simulink model "IID_nms_2Dmodel_inv"  (R2016b)
settings: Solver=ode3  StartTime=0.0  StopTime=tend  FixedStep=ts  RelTol=1e-3  EnableMultiTasking=on
InitFcn:
  | IID_runScripts_inv;
values from neighbouring files (symbols this model uses):
  DeltaThRef = 5e-3    (= 0.005)    [IID_nms_MechInit.m]    (also in nms_MechInit.m)
  MidDelay = 0.010    (= 0.01)    [IID_setCtrlPar.m]    (also in nms_MechInit.m = 0.005)
  ShortDelay = 0.005    [IID_setCtrlPar.m]    (also in nms_MechInit.m = 0.0025)
libraries: cpg_lib x18, simulink x11, simulink_extras x2
settings Model: SimulationMode=accelerator  Creator=Tycho  LastModifiedBy=brugtjh
settings DataIOCC: SignalLogging=off  SignalLoggingName=logout
settings OptimizationCC: LifeSpan=inf
settings DebuggingCC: AllowSymbolicDim=off  SFUnexpectedBacktrackingDiag=warning  SFNoUnconditionalDefaultTransitionDiag=warning  SFExecutionAtInitializationDiag=none
settings ModelReferenceCC: PropagateSignalLabelsOutOfModel=off
settings GRTTargetCC: TargetLangStandard=C89/C90 (ANSI)
settings ConfigComp: CovMetricSettings=dw  CovHtmlReporting=on  CovSaveCumulativeToWorkspaceVar=on  CovSaveSingleToWorkspaceVar=on  CovExternalEMLEnable=off

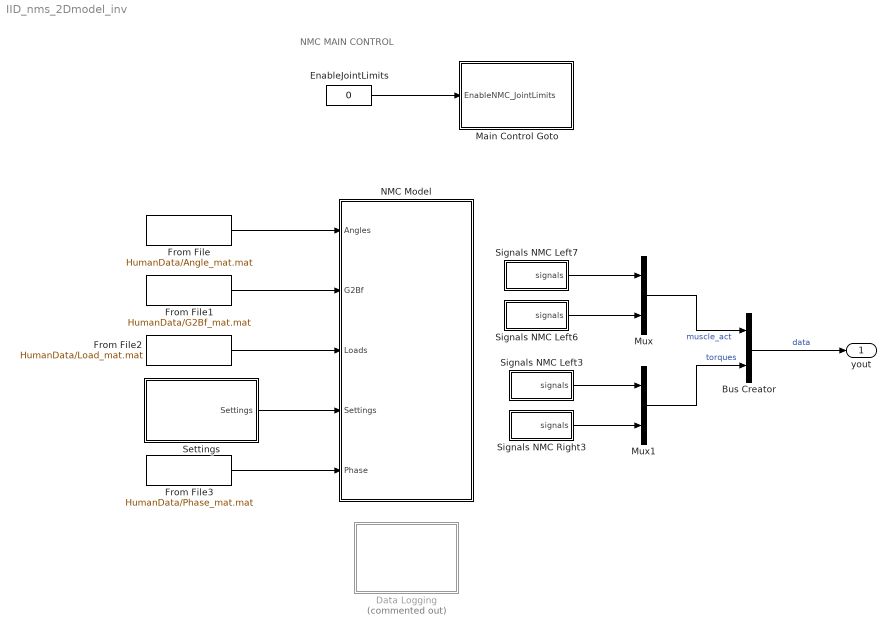
== system IID_nms_2Dmodel_inv ==
  note: NMC MAIN CONTROL
  Bus Creator : BusCreator  Inputs=2
  Data Logging : Subsystem  Commented=on
  EnableJointLimits : Constant  Value=0  OutDataTypeStr=double
      settings: OpenFcn=|
      | b = get_param(gcb,'value');
      | if (strcmp(b,'1')),
      |   set_param (gcb,'value','0');
      | else
      |   set_param(gcb,'value','1');
      | end;
  From File : FromFile  FileName=HumanData/Angle_mat.mat  SampleTime=0
  From File1 : FromFile  FileName=HumanData/G2Bf_mat.mat  SampleTime=0
  From File2 : FromFile  FileName=HumanData/Load_mat.mat  SampleTime=0
  From File3 : FromFile  FileName=HumanData/Phase_mat.mat  SampleTime=0
  Main Control Goto : Subsystem
  Mux : Mux  Inputs=2
  Mux1 : Mux  Inputs=2
  NMC Model : Subsystem
  Settings : Subsystem
  Signals NMC Left3 : Subsystem
  Signals NMC Left6 : Subsystem
  Signals NMC Left7 : Subsystem
  Signals NMC Right3 : Subsystem
  yout : Outport
  wires:
  Settings/1(Settings) -> NMC Model/4(Settings)
  EnableJointLimits/1 -> Main Control Goto/1(EnableNMC_JointLimits)
  From File/1 -> NMC Model/1(Angles)
  From File1/1 -> NMC Model/2(G2Bf)
  From File2/1 -> NMC Model/3(Loads)
  From File3/1 -> NMC Model/5(Phase)
  Signals NMC Left6/1(signals) -> Mux/2
  Signals NMC Left7/1(signals) -> Mux/1
  Signals NMC Left3/1(signals) -> Mux1/1
  Signals NMC Right3/1(signals) -> Mux1/2
  Mux/1 -> Bus Creator/1  "muscle_act"
  Mux1/1 -> Bus Creator/2  "torques"
  Bus Creator/1 -> yout/1  "data"

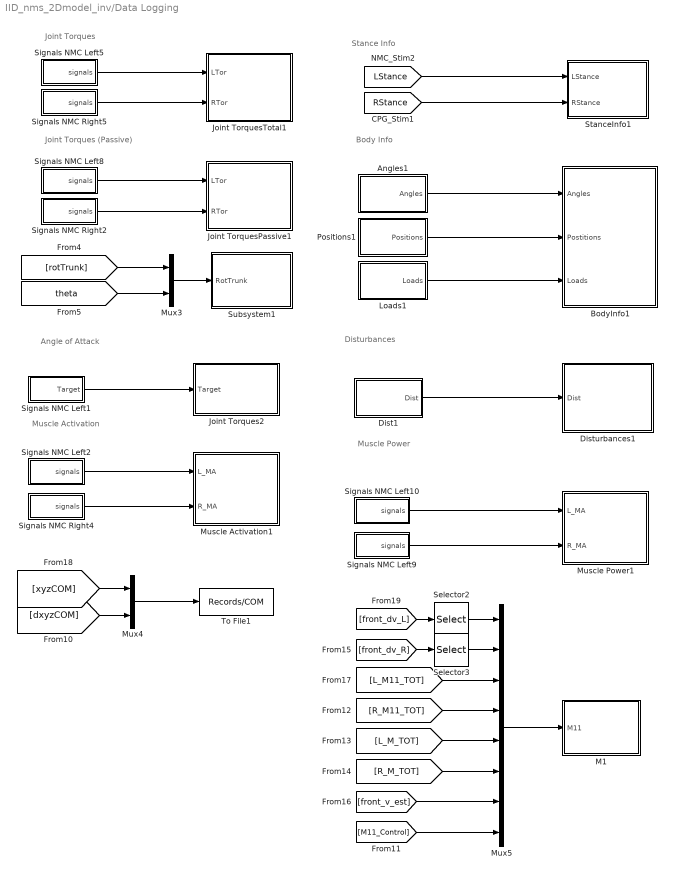
== system IID_nms_2Dmodel_inv/Data Logging ==
  note: Disturbances
  note: Stance Info
  note: Muscle Activation
  note: Joint Torques
  note: Angle of Attack
  note: Body Info
  note: Joint Torques (Passive)
  note: Muscle Power
  Angles1 : Subsystem
  BodyInfo1 : Subsystem
  Dist1 : Subsystem
  Disturbances1 : Subsystem
  Joint Torques2 : Subsystem
  Joint TorquesPassive1 : Subsystem
  Joint TorquesTotal1 : Subsystem
  Loads1 : Subsystem
  M1 : Subsystem
  Muscle Activation1 : Subsystem
  Muscle Power1 : Subsystem
  Mux3 : Mux  Inputs=2
  Mux4 : Mux  Inputs=2
  Mux5 : Mux  Inputs=8
  Positions1 : Subsystem
  Selector2 : Selector  InputPortWidth=2  IndexOptions=Index vector (dialog)  Indices=[2]  OutputSizes=1
  Selector3 : Selector  InputPortWidth=2  IndexOptions=Index vector (dialog)  Indices=[2]  OutputSizes=1
  Signals NMC Left1 : Subsystem
  Signals NMC Left10 : Subsystem
  Signals NMC Left2 : Subsystem
  Signals NMC Left5 : Subsystem
  Signals NMC Left8 : Subsystem
  Signals NMC Left9 : Subsystem
  Signals NMC Right2 : Subsystem
  Signals NMC Right4 : Subsystem
  Signals NMC Right5 : Subsystem
  StanceInfo1 : Subsystem
  Subsystem1 : Subsystem
  To File1 : ToFile  Filename=Records/COM
  wires:
  Dist1/1(Dist) -> Disturbances1/1(Dist)
  Signals NMC Right4/1(signals) -> Muscle Activation1/2(R_MA)
  Signals NMC Left2/1(signals) -> Muscle Activation1/1(L_MA)
  Signals NMC Left5/1(signals) -> Joint TorquesTotal1/1(LTor)
  Signals NMC Right5/1(signals) -> Joint TorquesTotal1/2(RTor)
  Angles1/1(Angles) -> BodyInfo1/1(Angles)
  Positions1/1(Positions) -> BodyInfo1/2(Postitions)
  [LStance] -> StanceInfo1/1(LStance)
  [RStance] -> StanceInfo1/2(RStance)
  Loads1/1(Loads) -> BodyInfo1/3(Loads)
  Signals NMC Left1/1(Target) -> Joint Torques2/1(Target)
  [rotTrunk] -> Mux3/1
  [theta] -> Mux3/2
  Signals NMC Left8/1(signals) -> Joint TorquesPassive1/1(LTor)
  Signals NMC Right2/1(signals) -> Joint TorquesPassive1/2(RTor)
  Signals NMC Left9/1(signals) -> Muscle Power1/2(R_MA)
  Signals NMC Left10/1(signals) -> Muscle Power1/1(L_MA)
  Mux3/1 -> Subsystem1/1(RotTrunk)
  [dxyzCOM] -> Mux4/2
  [xyzCOM] -> Mux4/1
  Mux4/1 -> To File1/1
  Selector2/1 -> Mux5/1
  [front_dv_L] -> Selector2/1
  [L_M_TOT] -> Mux5/5
  [R_M_TOT] -> Mux5/6
  [L_M11_TOT] -> Mux5/3
  [R_M11_TOT] -> Mux5/4
  [front_dv_R] -> Selector3/1
  Selector3/1 -> Mux5/2
  Mux5/1 -> M1/1(M11)
  [M11_Control] -> Mux5/8
  [front_v_est] -> Mux5/7

== system IID_nms_2Dmodel_inv/Main Control Goto ==
  EnableNMC_JointLimits : Inport
  tag scope: DisableNMC_JointLimitsIn=global
  wires:
  EnableNMC_JointLimits/1 -> [DisableNMC_JointLimitsIn]

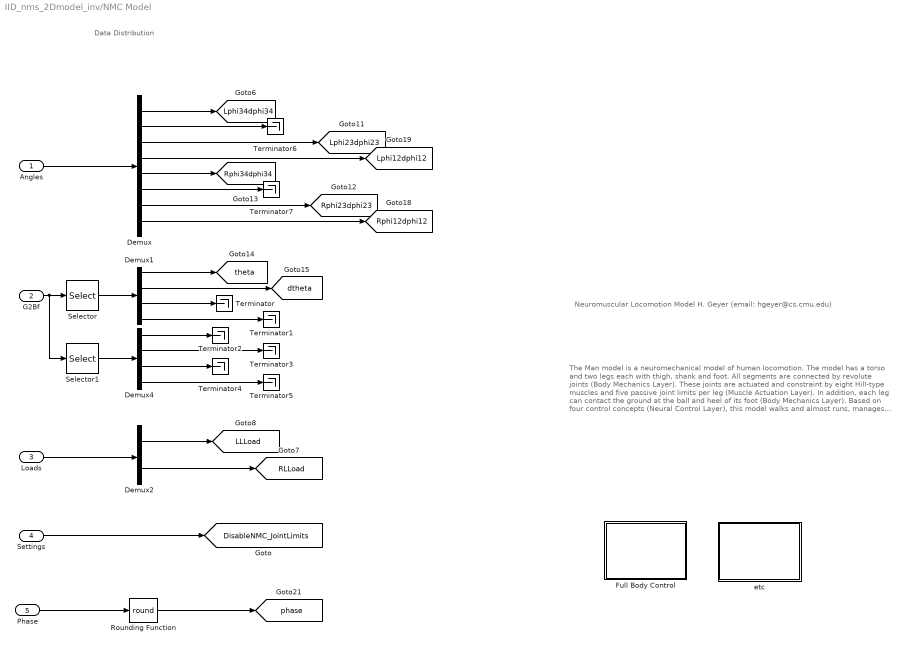
== system IID_nms_2Dmodel_inv/NMC Model ==
  note: Data Distribution
  note: The Man model is a neuromechanical model of human locomotion.
      | The model has a torso and two legs each with thigh, shank and
      | foot. All segments are connected by revolute joints (Body Mechanics
      | Layer). These joints are actuated and constraint by eight Hill-type
      | muscles and five passive joint limits per leg (Muscle Actuation Layer).
      | In addition, each leg can contact the ground at the ball and heel of
      | its foot (Body Mechanics Layer).
      |
      | Based on four control concepts (Neural Control Layer), this
      | model walks and almost runs, manages slopes and random ground
      | levels, and adapts to different surfaces.
  note: Neuromuscular Locomotion Model
      | H. Geyer
      | (email: hgeyer@cs.cmu.edu)
  Angles : Inport
  G2Bf : Inport  Port=2
  Loads : Inport  Port=3
  Settings : Inport  Port=4
  Phase : Inport  Port=5
  Demux : Demux  Outputs=8
  Demux1 : Demux
  Demux2 : Demux  Outputs=2
  Demux4 : Demux
  Full Body Control : Subsystem
  Rounding Function : Rounding  Operator=round
  Selector : Selector  InputPortWidth=12  IndexOptions=Index vector (dialog)  Indices=[1:4]  OutputSizes=1
  Selector1 : Selector  InputPortWidth=12  IndexOptions=Index vector (dialog)  Indices=[5:12]  OutputSizes=1
  Terminator{,1..7} (8 alike) : Terminator
  etc : Subsystem
  tag scope: DisableNMC_JointLimits=global, LLLoad=global, Lphi12dphi12=global, Lphi23dphi23=global, Lphi34dphi34=global, RLLoad=global, Rphi12dphi12=global, Rphi23dphi23=global, Rphi34dphi34=global, dtheta=global, phase=global, theta=global
  wires:
  Settings/1 -> [DisableNMC_JointLimits]
  Phase/1 -> Rounding Function/1
  Loads/1 -> Demux2/1
  G2Bf/1 -> Selector1/1, Selector/1
  Demux/4 -> [Lphi12dphi12]
  Demux/3 -> [Lphi23dphi23]
  Demux/2 -> Terminator6/1
  Demux/8 -> [Rphi12dphi12]
  Demux/7 -> [Rphi23dphi23]
  Demux/6 -> Terminator7/1
  Demux/5 -> [Rphi34dphi34]
  Demux/1 -> [Lphi34dphi34]
  Angles/1 -> Demux/1
  Demux1/4 -> Terminator1/1
  Demux1/3 -> Terminator/1
  Demux1/2 -> [dtheta]
  Demux1/1 -> [theta]
  Selector/1 -> Demux1/1
  Selector1/1 -> Demux4/1
  Rounding Function/1 -> [phase]
  Demux4/1 -> Terminator2/1
  Demux4/3 -> Terminator4/1
  Demux4/2 -> Terminator3/1
  Demux4/4 -> Terminator5/1
  Demux2/1 -> [LLLoad]
  Demux2/2 -> [RLLoad]

== system IID_nms_2Dmodel_inv/Settings ==
  Settings : Outport
  wires:
  [DisableNMC_JointLimitsIn] -> Settings/1

== system IID_nms_2Dmodel_inv/Signals NMC Left3 ==
  Mux : Mux
  signals : Outport
  wires:
  Mux/1 -> signals/1
  [LM34] -> Mux/1
  [LM23] -> Mux/3
  [LM12] -> Mux/4
  [LM34R] -> Mux/2

== system IID_nms_2Dmodel_inv/Signals NMC Left6 ==
  Mux : Mux  Inputs=7
  signals : Outport
  wires:
  Mux/1 -> signals/1
  [REnergyVAS] -> Mux/2
  [REnergyHFL] -> Mux/1
  [REnergyTA] -> Mux/3
  [REnergySOL] -> Mux/4
  [REnergyHAM] -> Mux/6
  [REnergyGAS] -> Mux/5
  [REnergyGLU] -> Mux/7

== system IID_nms_2Dmodel_inv/Signals NMC Left7 ==
  Mux : Mux  Inputs=7
  signals : Outport
  wires:
  Mux/1 -> signals/1
  [LEnergyVAS] -> Mux/2
  [LEnergyHFL] -> Mux/1
  [LEnergyTA] -> Mux/3
  [LEnergySOL] -> Mux/4
  [LEnergyHAM] -> Mux/6
  [LEnergyGAS] -> Mux/5
  [LEnergyGLU] -> Mux/7

== system IID_nms_2Dmodel_inv/Signals NMC Right3 ==
  Mux : Mux
  signals : Outport
  wires:
  Mux/1 -> signals/1
  [RM34] -> Mux/1
  [RM23] -> Mux/3
  [RM12] -> Mux/4
  [RM34R] -> Mux/2

== system IID_nms_2Dmodel_inv/Data Logging/Angles1 ==
  Constant : Constant  Value=zeros(2,1)
  Constant1 : Constant  Value=zeros(2,1)
  Mux : Mux  Inputs=8
  Angles : Outport
  wires:
  [Rphi12dphi12] -> Mux/8
  [Lphi34dphi34] -> Mux/1
  [Rphi23dphi23] -> Mux/7
  [Lphi23dphi23] -> Mux/3
  Constant1/1 -> Mux/6
  Constant/1 -> Mux/2
  [Lphi12dphi12] -> Mux/4
  [Rphi34dphi34] -> Mux/5
  Mux/1 -> Angles/1

== system IID_nms_2Dmodel_inv/Data Logging/BodyInfo1 ==
  Angles : Inport
  Postitions : Inport  Port=2
  Loads : Inport  Port=3
  Mux1 : Mux  Inputs=3
  To File8 : ToFile  Filename=Records/BodyInfo
  wires:
  Loads/1 -> Mux1/3
  Postitions/1 -> Mux1/2
  Mux1/1 -> To File8/1
  Angles/1 -> Mux1/1

== system IID_nms_2Dmodel_inv/Data Logging/Dist1 ==
  Dist : Outport
  wires:
  [xyzHAT_D_sag] -> Dist/1

== system IID_nms_2Dmodel_inv/Data Logging/Disturbances1 ==
  Dist : Inport
  To File21 : ToFile  Filename=Records/Disturbance
  wires:
  Dist/1 -> To File21/1

== system IID_nms_2Dmodel_inv/Data Logging/Joint Torques2 ==
  Target : Inport
  To File12 : ToFile  Filename=Records/TargetAngle
  wires:
  Target/1 -> To File12/1

== system IID_nms_2Dmodel_inv/Data Logging/Joint TorquesPassive1 ==
  LTor : Inport
  RTor : Inport  Port=2
  To File12 : ToFile  Filename=Records/L_Tor_Passive
  To File9 : ToFile  Filename=Records/R_Tor_Passvie
  wires:
  RTor/1 -> To File9/1
  LTor/1 -> To File12/1

== system IID_nms_2Dmodel_inv/Data Logging/Joint TorquesTotal1 ==
  LTor : Inport
  RTor : Inport  Port=2
  To File12 : ToFile  Filename=Records/L_Tor
  To File9 : ToFile  Filename=Records/R_Tor
  wires:
  LTor/1 -> To File12/1
  RTor/1 -> To File9/1

== system IID_nms_2Dmodel_inv/Data Logging/Loads1 ==
  Mux : Mux  Inputs=2
  Loads : Outport
  wires:
  [LLLoad] -> Mux/2
  [RLLoad] -> Mux/1
  Mux/1 -> Loads/1

== system IID_nms_2Dmodel_inv/Data Logging/M1 ==
  M11 : Inport
  To File2 : ToFile  Filename=Records/M11
  wires:
  M11/1 -> To File2/1

== system IID_nms_2Dmodel_inv/Data Logging/Muscle Activation1 ==
  L_MA : Inport
  R_MA : Inport  Port=2
  To File1 : ToFile  Filename=Records/R_MA
  To File5 : ToFile  Filename=Records/L_MA
  wires:
  L_MA/1 -> To File5/1
  R_MA/1 -> To File1/1

== system IID_nms_2Dmodel_inv/Data Logging/Muscle Power1 ==
  L_MA : Inport
  R_MA : Inport  Port=2
  To File1 : ToFile  Filename=Records/R_Power
  To File5 : ToFile  Filename=Records/L_Power
  wires:
  L_MA/1 -> To File5/1
  R_MA/1 -> To File1/1

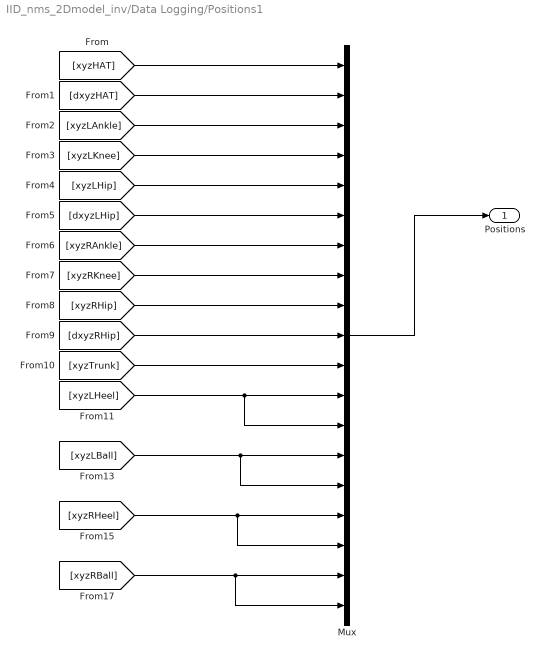
== system IID_nms_2Dmodel_inv/Data Logging/Positions1 ==
  Mux : Mux  Inputs=19
  Positions : Outport
  wires:
  [xyzRBall] -> Mux/19, Mux/18
  [xyzRHeel] -> Mux/17, Mux/16
  [xyzLBall] -> Mux/15, Mux/14
  [xyzLHeel] -> Mux/13, Mux/12
  [xyzTrunk] -> Mux/11
  [dxyzHAT] -> Mux/2
  [xyzHAT] -> Mux/1
  [dxyzRHip] -> Mux/10
  [xyzRHip] -> Mux/9
  [xyzLAnkle] -> Mux/3
  [xyzRKnee] -> Mux/8
  [dxyzLHip] -> Mux/6
  [xyzLHip] -> Mux/5
  [xyzLKnee] -> Mux/4
  [xyzRAnkle] -> Mux/7
  Mux/1 -> Positions/1

== system IID_nms_2Dmodel_inv/Data Logging/Signals NMC Left1 ==
  Mux : Mux
  Target : Outport
  wires:
  Mux/1 -> Target/1
  [Lalpha_tgt] -> Mux/1
  [LhipR_tgt] -> Mux/3
  [RhipR_tgt] -> Mux/4
  [Ralpha_tgt] -> Mux/2

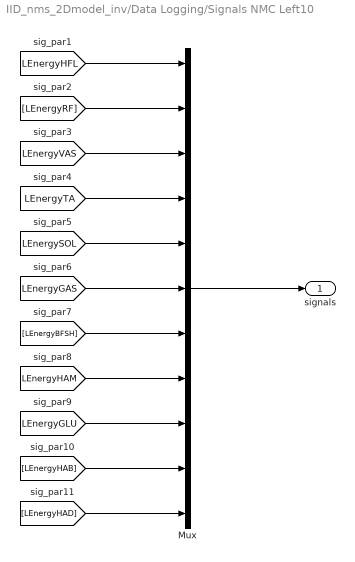
== system IID_nms_2Dmodel_inv/Data Logging/Signals NMC Left10 ==
  Mux : Mux  Inputs=11
  signals : Outport
  wires:
  [LEnergyRF] -> Mux/2
  [LEnergyTA] -> Mux/4
  [LEnergyGAS] -> Mux/6
  [LEnergyHAM] -> Mux/8
  [LEnergyHAB] -> Mux/10
  [LEnergySOL] -> Mux/5
  [LEnergyHAD] -> Mux/11
  [LEnergyBFSH] -> Mux/7
  [LEnergyVAS] -> Mux/3
  [LEnergyGLU] -> Mux/9
  [LEnergyHFL] -> Mux/1
  Mux/1 -> signals/1

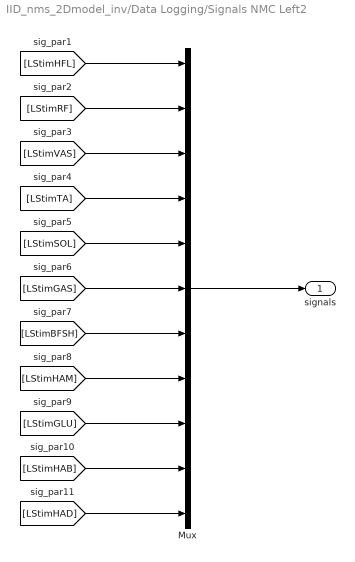
== system IID_nms_2Dmodel_inv/Data Logging/Signals NMC Left2 ==
  Mux : Mux  Inputs=11
  signals : Outport
  wires:
  [LStimRF] -> Mux/2
  [LStimTA] -> Mux/4
  [LStimGAS] -> Mux/6
  [LStimHAM] -> Mux/8
  [LStimHAB] -> Mux/10
  [LStimSOL] -> Mux/5
  [LStimHAD] -> Mux/11
  [LStimBFSH] -> Mux/7
  [LStimVAS] -> Mux/3
  [LStimGLU] -> Mux/9
  [LStimHFL] -> Mux/1
  Mux/1 -> signals/1

== system IID_nms_2Dmodel_inv/Data Logging/Signals NMC Left5 ==
  Mux : Mux
  signals : Outport
  wires:
  [LM34R] -> Mux/2
  [LM12] -> Mux/4
  [LM23] -> Mux/3
  [LM34] -> Mux/1
  Mux/1 -> signals/1

== system IID_nms_2Dmodel_inv/Data Logging/Signals NMC Left8 ==
  Mux : Mux
  signals : Outport
  wires:
  Mux/1 -> signals/1
  [LHipStop] -> Mux/1
  [LKneeStop] -> Mux/3
  [LAnkleStop] -> Mux/4
  [LHipRStop] -> Mux/2

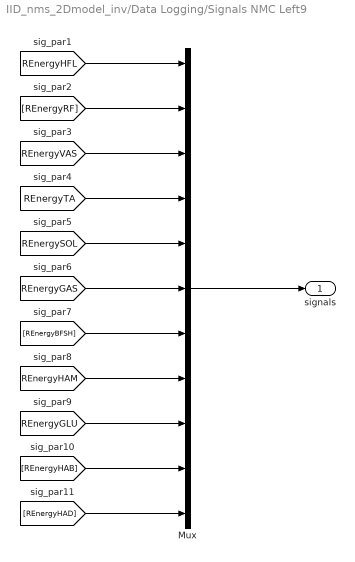
== system IID_nms_2Dmodel_inv/Data Logging/Signals NMC Left9 ==
  Mux : Mux  Inputs=11
  signals : Outport
  wires:
  Mux/1 -> signals/1
  [REnergyHFL] -> Mux/1
  [REnergyGLU] -> Mux/9
  [REnergyVAS] -> Mux/3
  [REnergyBFSH] -> Mux/7
  [REnergyHAD] -> Mux/11
  [REnergySOL] -> Mux/5
  [REnergyHAB] -> Mux/10
  [REnergyHAM] -> Mux/8
  [REnergyGAS] -> Mux/6
  [REnergyTA] -> Mux/4
  [REnergyRF] -> Mux/2

== system IID_nms_2Dmodel_inv/Data Logging/Signals NMC Right2 ==
  Mux : Mux
  signals : Outport
  wires:
  Mux/1 -> signals/1
  [RHipStop] -> Mux/1
  [RKneeStop] -> Mux/3
  [RAnkleStop] -> Mux/4
  [RHipStopR] -> Mux/2

== system IID_nms_2Dmodel_inv/Data Logging/Signals NMC Right4 ==
  Mux : Mux  Inputs=11
  signals : Outport
  wires:
  Mux/1 -> signals/1
  [RStimHFL] -> Mux/1
  [RStimGLU] -> Mux/9
  [RStimVAS] -> Mux/3
  [RStimBFSH] -> Mux/7
  [RStimHAD] -> Mux/11
  [RStimSOL] -> Mux/5
  [RStimHAB] -> Mux/10
  [RStimHAM] -> Mux/8
  [RStimGAS] -> Mux/6
  [RStimTA] -> Mux/4
  [RStimRF] -> Mux/2

== system IID_nms_2Dmodel_inv/Data Logging/Signals NMC Right5 ==
  Mux : Mux
  signals : Outport
  wires:
  [RM34R] -> Mux/2
  [RM12] -> Mux/4
  [RM23] -> Mux/3
  [RM34] -> Mux/1
  Mux/1 -> signals/1

== system IID_nms_2Dmodel_inv/Data Logging/StanceInfo1 ==
  LStance : Inport
  RStance : Inport  Port=2
  Mux4 : Mux  Inputs=2
  To File4 : ToFile  Filename=Records/StanceSig
  wires:
  LStance/1 -> Mux4/1
  RStance/1 -> Mux4/2
  Mux4/1 -> To File4/1

== system IID_nms_2Dmodel_inv/Data Logging/Subsystem1 ==
  RotTrunk : Inport
  To File8 : ToFile  Filename=Records/rotTrunk
  wires:
  RotTrunk/1 -> To File8/1

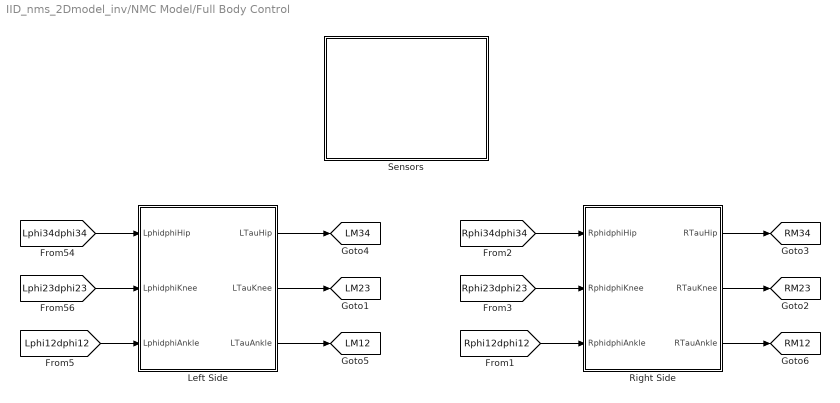
== system IID_nms_2Dmodel_inv/NMC Model/Full Body Control ==
  Left Side : Subsystem
  Right Side : Subsystem
  Sensors : Subsystem
  tag scope: LM12=global, LM23=global, LM34=global, RM12=global, RM23=global, RM34=global
  wires:
  [Lphi34dphi34] -> Left Side/1(LphidphiHip)
  [Lphi23dphi23] -> Left Side/2(LphidphiKnee)
  Left Side/1(LTauHip) -> [LM34]
  Left Side/2(LTauKnee) -> [LM23]
  Left Side/3(LTauAnkle) -> [LM12]
  [Lphi12dphi12] -> Left Side/3(LphidphiAnkle)
  [Rphi34dphi34] -> Right Side/1(RphidphiHip)
  [Rphi23dphi23] -> Right Side/2(RphidphiKnee)
  [Rphi12dphi12] -> Right Side/3(RphidphiAnkle)
  Right Side/1(RTauHip) -> [RM34]
  Right Side/2(RTauKnee) -> [RM23]
  Right Side/3(RTauAnkle) -> [RM12]

== system IID_nms_2Dmodel_inv/NMC Model/etc ==
  note: Fall detection
      | (stop simulation)
  Abs3 : Abs
  Compare To Constant2 : simulink/Logic and Bit Operations/Compare To Constant  relop=>  const=60*pi/180  OutDataTypeStr=boolean
  Stop Simulation : Stop
  wires:
  Compare To Constant2/1 -> Stop Simulation/1
  Abs3/1 -> Compare To Constant2/1
  [theta] -> Abs3/1

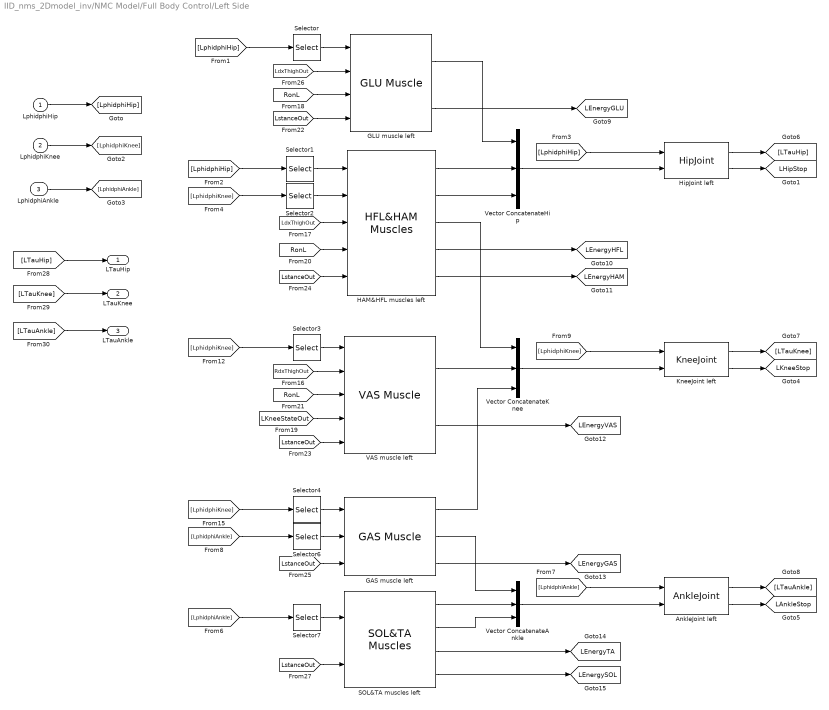
== system IID_nms_2Dmodel_inv/NMC Model/Full Body Control/Left Side ==
  LphidphiHip : Inport
  LphidphiKnee : Inport  Port=2
  LphidphiAnkle : Inport  Port=3
  AnkleJoint left : cpg_lib/AnkleJoint
  GAS muscle left : cpg_lib/GAS Muscle
  GLU muscle left : cpg_lib/GLU Muscle
  HAM&HFL muscles left : cpg_lib/HFL&HAM Muscles
  HipJoint left : cpg_lib/HipJoint
  KneeJoint left : cpg_lib/KneeJoint
  SOL&TA muscles left : cpg_lib/SOL&TA Muscles
  Selector{,1..4,6..7} (7 alike) : Selector  InputPortWidth=2  IndexOptions=Index vector (dialog)  Indices=[1 ]  OutputSizes=1
  VAS muscle left : cpg_lib/VAS Muscle
  Vector ConcatenateAnkle : Concatenate  NumInputs=3
  Vector ConcatenateHip : Concatenate  NumInputs=3
  Vector ConcatenateKnee : Concatenate  NumInputs=3
  LTauHip : Outport
  LTauKnee : Outport  Port=2
  LTauAnkle : Outport  Port=3
  tag scope: LAnkleStop=global, LEnergyGAS=global, LEnergyGLU=global, LEnergyHAM=global, LEnergyHFL=global, LEnergySOL=global, LEnergyTA=global, LEnergyVAS=global, LHipStop=global, LKneeStop=global
  wires:
  GAS muscle left/2 -> Vector ConcatenateAnkle/1
  Vector ConcatenateHip/1 -> HipJoint left/2
  [LphidphiKnee] -> KneeJoint left/1
  Selector1/1 -> HAM&HFL muscles left/1
  Selector4/1 -> GAS muscle left/1
  [RdxThighOut] -> VAS muscle left/2
  SOL&TA muscles left/2 -> Vector ConcatenateAnkle/3
  Selector7/1 -> SOL&TA muscles left/1
  Vector ConcatenateAnkle/1 -> AnkleJoint left/2
  Vector ConcatenateKnee/1 -> KneeJoint left/2
  SOL&TA muscles left/1 -> Vector ConcatenateAnkle/2
  Selector3/1 -> VAS muscle left/1
  Selector6/1 -> GAS muscle left/2
  VAS muscle left/1 -> Vector ConcatenateKnee/2
  [LphidphiAnkle] -> AnkleJoint left/1
  GAS muscle left/1 -> Vector ConcatenateKnee/3
  HAM&HFL muscles left/1 -> Vector ConcatenateHip/2
  GLU muscle left/1 -> Vector ConcatenateHip/1
  [LstanceOut] -> HAM&HFL muscles left/5
  [RonL] -> VAS muscle left/3
  [LphidphiKnee] -> Selector3/1
  [LphidphiKnee] -> Selector4/1
  [RonL] -> HAM&HFL muscles left/4
  [LKneeStateOut] -> VAS muscle left/4
  HAM&HFL muscles left/3 -> Vector ConcatenateKnee/1
  Selector/1 -> GLU muscle left/1
  [LstanceOut] -> GAS muscle left/3
  [LphidphiAnkle] -> Selector7/1
  [LstanceOut] -> SOL&TA muscles left/2
  HAM&HFL muscles left/2 -> Vector ConcatenateHip/3
  Selector2/1 -> HAM&HFL muscles left/2
  [LphidphiAnkle] -> Selector6/1
  [LphidphiHip] -> Selector1/1
  [LstanceOut] -> VAS muscle left/5
  [LphidphiHip] -> Selector/1
  [LphidphiHip] -> HipJoint left/1
  [LphidphiKnee] -> Selector2/1
  HipJoint left/1 -> [LTauHip]
  KneeJoint left/1 -> [LTauKnee]
  AnkleJoint left/1 -> [LTauAnkle]
  [LdxThighOut] -> GLU muscle left/2
  [LstanceOut] -> GLU muscle left/4
  [RonL] -> GLU muscle left/3
  [LdxThighOut] -> HAM&HFL muscles left/3
  LphidphiHip/1 -> [LphidphiHip]
  LphidphiKnee/1 -> [LphidphiKnee]
  LphidphiAnkle/1 -> [LphidphiAnkle]
  [LTauHip] -> LTauHip/1
  [LTauKnee] -> LTauKnee/1
  [LTauAnkle] -> LTauAnkle/1
  HipJoint left/2 -> [LHipStop]
  KneeJoint left/2 -> [LKneeStop]
  AnkleJoint left/2 -> [LAnkleStop]
  GLU muscle left/2 -> [LEnergyGLU]
  HAM&HFL muscles left/4 -> [LEnergyHFL]
  HAM&HFL muscles left/5 -> [LEnergyHAM]
  VAS muscle left/2 -> [LEnergyVAS]
  GAS muscle left/3 -> [LEnergyGAS]
  SOL&TA muscles left/3 -> [LEnergyTA]
  SOL&TA muscles left/4 -> [LEnergySOL]

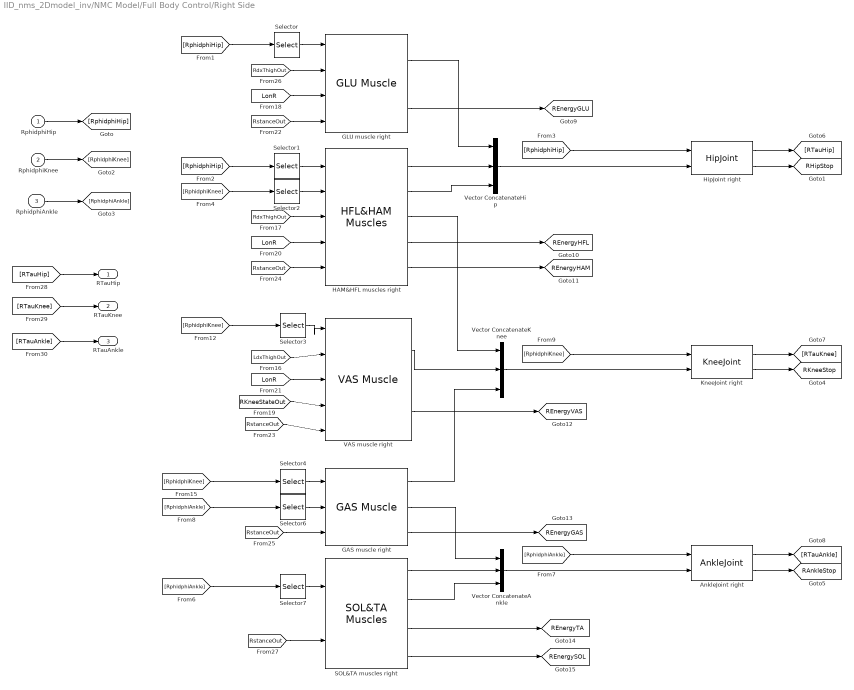
== system IID_nms_2Dmodel_inv/NMC Model/Full Body Control/Right Side ==
  RphidphiHip : Inport
  RphidphiKnee : Inport  Port=2
  RphidphiAnkle : Inport  Port=3
  AnkleJoint right : cpg_lib/AnkleJoint
  GAS muscle right : cpg_lib/GAS Muscle
  GLU muscle right : cpg_lib/GLU Muscle
  HAM&HFL muscles right : cpg_lib/HFL&HAM Muscles
  HipJoint right : cpg_lib/HipJoint
  KneeJoint right : cpg_lib/KneeJoint
  SOL&TA muscles right : cpg_lib/SOL&TA Muscles
  Selector{,1..4,6..7} (7 alike) : Selector  InputPortWidth=2  IndexOptions=Index vector (dialog)  Indices=[1 ]  OutputSizes=1
  VAS muscle right : cpg_lib/VAS Muscle
  Vector ConcatenateAnkle : Concatenate  NumInputs=3
  Vector ConcatenateHip : Concatenate  NumInputs=3
  Vector ConcatenateKnee : Concatenate  NumInputs=3
  RTauHip : Outport
  RTauKnee : Outport  Port=2
  RTauAnkle : Outport  Port=3
  tag scope: RAnkleStop=global, REnergyGAS=global, REnergyGLU=global, REnergyHAM=global, REnergyHFL=global, REnergySOL=global, REnergyTA=global, REnergyVAS=global, RHipStop=global, RKneeStop=global
  wires:
  GAS muscle right/2 -> Vector ConcatenateAnkle/1
  Vector ConcatenateHip/1 -> HipJoint right/2
  [RphidphiKnee] -> KneeJoint right/1
  Selector1/1 -> HAM&HFL muscles right/1
  Selector4/1 -> GAS muscle right/1
  [LdxThighOut] -> VAS muscle right/2
  SOL&TA muscles right/2 -> Vector ConcatenateAnkle/3
  Selector7/1 -> SOL&TA muscles right/1
  Vector ConcatenateAnkle/1 -> AnkleJoint right/2
  Vector ConcatenateKnee/1 -> KneeJoint right/2
  SOL&TA muscles right/1 -> Vector ConcatenateAnkle/2
  Selector3/1 -> VAS muscle right/1
  Selector6/1 -> GAS muscle right/2
  VAS muscle right/1 -> Vector ConcatenateKnee/2
  [RphidphiAnkle] -> AnkleJoint right/1
  GAS muscle right/1 -> Vector ConcatenateKnee/3
  HAM&HFL muscles right/1 -> Vector ConcatenateHip/2
  GLU muscle right/1 -> Vector ConcatenateHip/1
  [LonR] -> VAS muscle right/3
  [RphidphiKnee] -> Selector3/1
  [RphidphiKnee] -> Selector4/1
  [RKneeStateOut] -> VAS muscle right/4
  HAM&HFL muscles right/3 -> Vector ConcatenateKnee/1
  Selector/1 -> GLU muscle right/1
  [RstanceOut] -> GAS muscle right/3
  [RphidphiAnkle] -> Selector7/1
  [RstanceOut] -> SOL&TA muscles right/2
  HAM&HFL muscles right/2 -> Vector ConcatenateHip/3
  Selector2/1 -> HAM&HFL muscles right/2
  [RphidphiAnkle] -> Selector6/1
  [RphidphiHip] -> Selector1/1
  [RstanceOut] -> VAS muscle right/5
  [RphidphiHip] -> Selector/1
  [RphidphiHip] -> HipJoint right/1
  [RphidphiKnee] -> Selector2/1
  HipJoint right/1 -> [RTauHip]
  KneeJoint right/1 -> [RTauKnee]
  AnkleJoint right/1 -> [RTauAnkle]
  [RdxThighOut] -> GLU muscle right/2
  [LonR] -> GLU muscle right/3
  [RstanceOut] -> GLU muscle right/4
  [RdxThighOut] -> HAM&HFL muscles right/3
  [LonR] -> HAM&HFL muscles right/4
  [RstanceOut] -> HAM&HFL muscles right/5
  RphidphiHip/1 -> [RphidphiHip]
  RphidphiKnee/1 -> [RphidphiKnee]
  RphidphiAnkle/1 -> [RphidphiAnkle]
  [RTauHip] -> RTauHip/1
  [RTauKnee] -> RTauKnee/1
  [RTauAnkle] -> RTauAnkle/1
  HipJoint right/2 -> [RHipStop]
  KneeJoint right/2 -> [RKneeStop]
  AnkleJoint right/2 -> [RAnkleStop]
  GLU muscle right/2 -> [REnergyGLU]
  HAM&HFL muscles right/4 -> [REnergyHFL]
  HAM&HFL muscles right/5 -> [REnergyHAM]
  VAS muscle right/2 -> [REnergyVAS]
  SOL&TA muscles right/3 -> [REnergyTA]
  SOL&TA muscles right/4 -> [REnergySOL]
  GAS muscle right/3 -> [REnergyGAS]

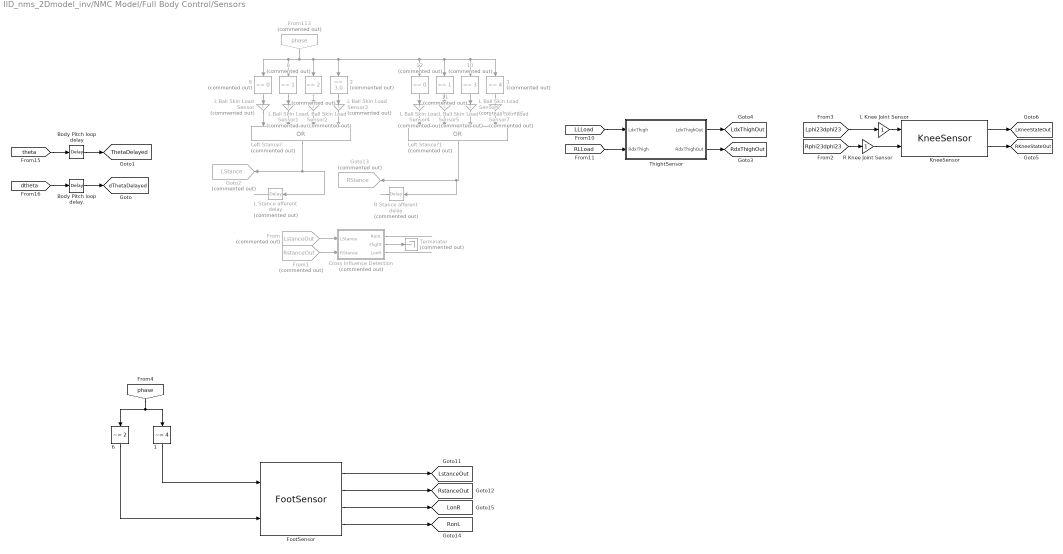
== system IID_nms_2Dmodel_inv/NMC Model/Full Body Control/Sensors ==
  " 1" : simulink/Logic and Bit Operations/Compare To Constant  relop=~=  const=4  OutDataTypeStr=boolean
  " 2" : simulink/Logic and Bit Operations/Compare To Constant  Commented=on  relop===  const=3.0  OutDataTypeStr=boolean
  " 3" : simulink/Logic and Bit Operations/Compare To Constant  Commented=on  relop===  const=4  OutDataTypeStr=boolean
  10 : simulink/Logic and Bit Operations/Compare To Constant  Commented=on  relop===  const=3  OutDataTypeStr=boolean
  11 : simulink/Logic and Bit Operations/Compare To Constant  Commented=on  relop===  const=1  OutDataTypeStr=boolean
  12 : simulink/Logic and Bit Operations/Compare To Constant  Commented=on  relop===  const=0  OutDataTypeStr=boolean
  6 : simulink/Logic and Bit Operations/Compare To Constant  relop=~=  const=2  OutDataTypeStr=boolean
  7 : simulink/Logic and Bit Operations/Compare To Constant  Commented=on  relop===  const=2  OutDataTypeStr=boolean
  8 : simulink/Logic and Bit Operations/Compare To Constant  Commented=on  relop===  const=1  OutDataTypeStr=boolean
  9 : simulink/Logic and Bit Operations/Compare To Constant  Commented=on  relop===  const=0  OutDataTypeStr=boolean
  Body Pitch loop delay : TransportDelay  DelayTime=ShortDelay
  Body Pitch loop delay. : TransportDelay  DelayTime=ShortDelay
  Cross Influence Detection : Subsystem  Commented=on
  FootSensor : cpg_lib/FootSensor
  From : From  Commented=on  GotoTag=LstanceOut  TagVisibility=global
  From1 : From  Commented=on  GotoTag=RstanceOut  TagVisibility=global
  From113 : From  Commented=on  GotoTag=phase  TagVisibility=global
      settings: CloseFcn=tagdialog Close
  Goto13 : Goto  Commented=on  GotoTag=RStance  TagVisibility=global
  Goto2 : Goto  Commented=on  GotoTag=LStance  TagVisibility=global
  KneeSensor : cpg_lib/KneeSensor
  L Ball Skin Load Sensor{,1..7} (8 alike) : Gain  Commented=on
  L Knee Joint Sensor : Gain
  L Stance afferent delay : TransportDelay  Commented=on  DelayTime=MidDelay
  Left Stance? : Logic  Commented=on  Operator=OR  Inputs=4  AllPortsSameDT=off
  Left Stance?1 : Logic  Commented=on  Operator=OR  Inputs=4  AllPortsSameDT=off
  R Knee Joint Sensor : Gain
  R Stance afferent delay : TransportDelay  Commented=on  DelayTime=MidDelay
  Terminator : Terminator  Commented=on
  ThightSensor : Subsystem
  tag scope: LKneeStateOut=global, LdxThighOut=global, LonR=global, LstanceOut=global, RKneeStateOut=global, RdxThighOut=global, RonL=global, RstanceOut=global, ThetaDelayed=global, dThetaDelayed=global
  wires:
  ThightSensor/2(RdxThighOut) -> [RdxThighOut]
  [RLLoad] -> ThightSensor/2(RdxThigh)
  ThightSensor/1(LdxThighOut) -> [LdxThighOut]
  [LLLoad] -> ThightSensor/1(LdxThigh)
  L Knee Joint Sensor/1 -> KneeSensor/1
  R Knee Joint Sensor/1 -> KneeSensor/2
  KneeSensor/1 -> [LKneeStateOut]
  KneeSensor/2 -> [RKneeStateOut]
  Body Pitch loop delay./1 -> [dThetaDelayed]
  Body Pitch loop delay/1 -> [ThetaDelayed]
  [theta] -> Body Pitch loop delay/1
  [dtheta] -> Body Pitch loop delay./1
  From/1 -> Cross Influence Detection/1(LStance)
  From1/1 -> Cross Influence Detection/2(RStance)
  9/1 -> L Ball Skin Load Sensor/1
  8/1 -> L Ball Skin Load Sensor1/1
  7/1 -> L Ball Skin Load Sensor2/1
  " 2"/1 -> L Ball Skin Load Sensor3/1
  12/1 -> L Ball Skin Load Sensor4/1
  11/1 -> L Ball Skin Load Sensor5/1
  10/1 -> L Ball Skin Load Sensor6/1
  " 3"/1 -> L Ball Skin Load Sensor7/1
  From113/1 -> " 3"/1, 10/1, 11/1, 12/1, " 2"/1, 7/1, 9/1, 8/1
  Cross Influence Detection/1(RonL) -> ?
  Cross Influence Detection/3(LonR) -> ?
  Cross Influence Detection/2(Flight) -> Terminator/1
  [Rphi23dphi23] -> R Knee Joint Sensor/1
  [Lphi23dphi23] -> L Knee Joint Sensor/1
  L Stance afferent delay/1 -> ?
  R Stance afferent delay/1 -> ?
  Left Stance?/1 -> L Stance afferent delay/1, Goto2/1
  Left Stance?1/1 -> Goto13/1, R Stance afferent delay/1
  L Ball Skin Load Sensor/1 -> Left Stance?/1
  L Ball Skin Load Sensor1/1 -> Left Stance?/2
  L Ball Skin Load Sensor2/1 -> Left Stance?/3
  L Ball Skin Load Sensor3/1 -> Left Stance?/4
  L Ball Skin Load Sensor4/1 -> Left Stance?1/1
  L Ball Skin Load Sensor5/1 -> Left Stance?1/2
  L Ball Skin Load Sensor6/1 -> Left Stance?1/3
  L Ball Skin Load Sensor7/1 -> Left Stance?1/4
  " 1"/1 -> FootSensor/1
  [phase] -> " 1"/1, 6/1
  6/1 -> FootSensor/2
  FootSensor/3 -> [LonR]
  FootSensor/4 -> [RonL]
  FootSensor/2 -> [RstanceOut]
  FootSensor/1 -> [LstanceOut]

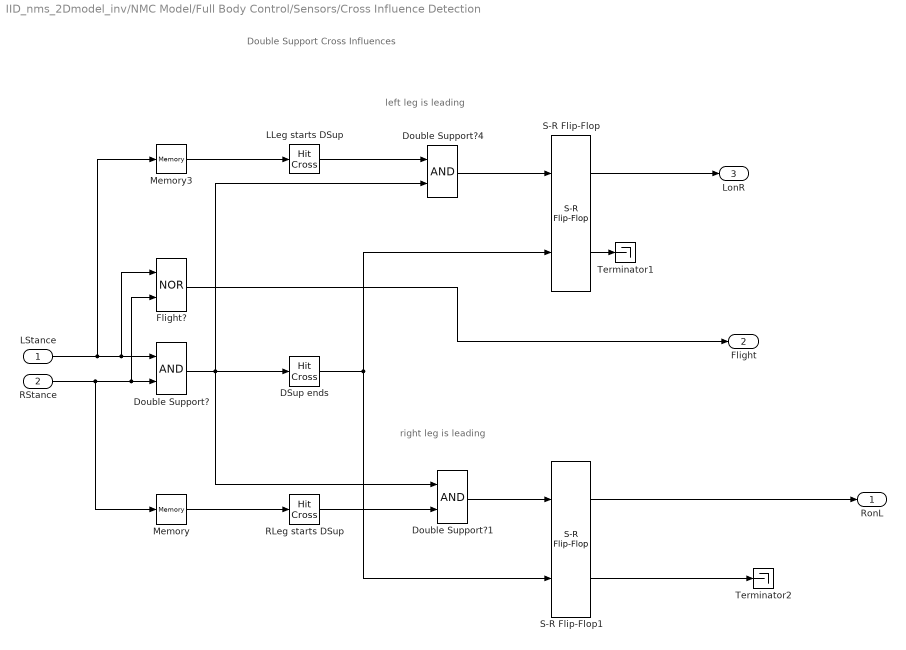
== system IID_nms_2Dmodel_inv/NMC Model/Full Body Control/Sensors/Cross Influence Detection ==
  note: Double Support Cross Influences
  note: right leg is leading
  note: left leg is leading
  LStance : Inport  OutDataTypeStr=double
  RStance : Inport  Port=2  OutDataTypeStr=double
  DSup ends : HitCross  HitCrossingOffset=0.5  HitCrossingDirection=falling  ZeroCross=off
  Double Support? : Logic  AllPortsSameDT=off
  Double Support?1 : Logic  AllPortsSameDT=off
  Double Support?4 : Logic  AllPortsSameDT=off
  Flight? : Logic  Operator=NOR  AllPortsSameDT=off
  LLeg starts DSup : HitCross  HitCrossingOffset=0.5  HitCrossingDirection=rising  ZeroCross=off
  Memory : Memory
  Memory3 : Memory
  RLeg starts DSup : HitCross  HitCrossingOffset=0.5  HitCrossingDirection=rising  ZeroCross=off
  S-R Flip-Flop : simulink_extras/Flip Flops/S-R Flip-Flop  initial_condition=0
  S-R Flip-Flop1 : simulink_extras/Flip Flops/S-R Flip-Flop  initial_condition=0
  Terminator1 : Terminator
  Terminator2 : Terminator
  RonL : Outport  OutDataTypeStr=double
  Flight : Outport  Port=2  OutDataTypeStr=double
  LonR : Outport  Port=3  OutDataTypeStr=double
  wires:
  RLeg starts DSup/1 -> Double Support?1/2
  S-R Flip-Flop/2 -> Terminator1/1
  S-R Flip-Flop1/2 -> Terminator2/1
  LStance/1 -> Memory3/1, Double Support?/1, Flight?/1
  LLeg starts DSup/1 -> Double Support?4/1
  RStance/1 -> Double Support?/2, Flight?/2, Memory/1
  Flight?/1 -> Flight/1
  Double Support?/1 -> DSup ends/1, Double Support?1/1, Double Support?4/2
  Memory/1 -> RLeg starts DSup/1
  Memory3/1 -> LLeg starts DSup/1
  DSup ends/1 -> S-R Flip-Flop/2, S-R Flip-Flop1/2
  Double Support?4/1 -> S-R Flip-Flop/1
  Double Support?1/1 -> S-R Flip-Flop1/1
  S-R Flip-Flop/1 -> LonR/1
  S-R Flip-Flop1/1 -> RonL/1

== system IID_nms_2Dmodel_inv/NMC Model/Full Body Control/Sensors/ThightSensor ==
  note: Body Mechanics Layer Interface
      | (Thigh Body Load Sensors)
  LdxThigh : Inport
  RdxThigh : Inport  Port=2
  FB Gain1 : Gain  Gain=DeltaThRef  SaturateOnIntegerOverflow=on  OutDataTypeStr=Inherit: Same as input  ParamDataTypeStr=Inherit: Same as input
  FB Gain2 : Gain  Gain=DeltaThRef  SaturateOnIntegerOverflow=on  OutDataTypeStr=Inherit: Same as input  ParamDataTypeStr=Inherit: Same as input
  L Thigh afferent delay : TransportDelay  DelayTime=ShortDelay
  R Thigh afferent delay : TransportDelay  DelayTime=ShortDelay
  LdxThighOut : Outport
  RdxThighOut : Outport  Port=2
  wires:
  L Thigh afferent delay/1 -> FB Gain1/1
  LdxThigh/1 -> L Thigh afferent delay/1
  RdxThigh/1 -> R Thigh afferent delay/1
  R Thigh afferent delay/1 -> FB Gain2/1
  FB Gain1/1 -> LdxThighOut/1
  FB Gain2/1 -> RdxThighOut/1
